simulink model "kepler_sgp4_test"  (Simulink 6.2)
settings: Solver=ode45  StartTime=0.0  StopTime=59516  RelTol=1e-3
undefined symbols (not defined in the file): onboardorbit, ONBOARDorbitECI
libraries: components_lib x4, simulink x2, sgp4_igrf_lib x2
settings Model: Creator=esch00  LastModifiedBy=rals
settings OptimizationCC: BlockReduction=off  BooleanDataType=off  InlineInvariantSignals=on
settings DebuggingCC: CheckSSInitialOutputMsg=off
settings HardwareCC: TargetUnknown=on

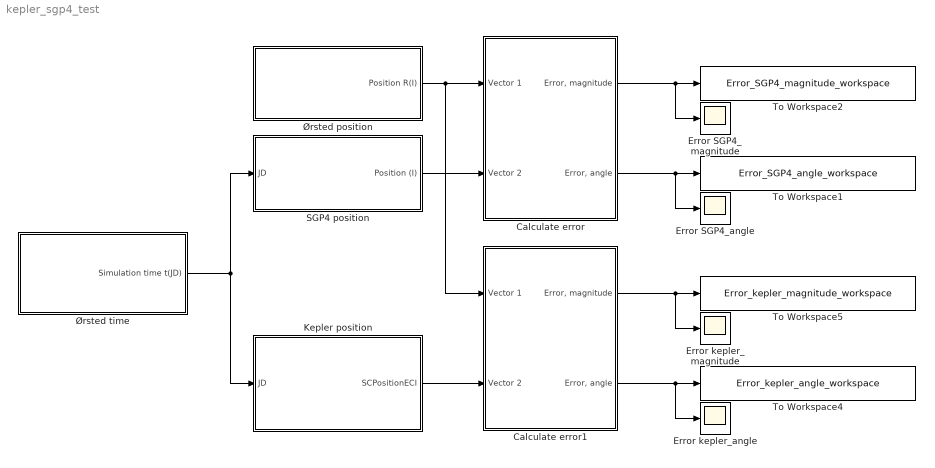
== system kepler_sgp4_test ==
  Calculate error : Subsystem
  Calculate error1 : Subsystem
  Error SGP4_angle : Scope
      settings: YMin=0  YMax=30000  SaveName=SGP4error1  DataFormat=Structure
  Error SGP4_magnitude : Scope
      settings: YMin=0  YMax=30000  SaveName=SGP4error  DataFormat=Structure
  Error kepler_angle : Scope
      settings: YMin=0  YMax=30000  SaveName=SGP4error2  DataFormat=Structure
  Error kepler_magnitude : Scope
      settings: YMin=0  YMax=30000  SaveName=SGP4error3  DataFormat=Structure
  Kepler position : Subsystem  AncestorBlock=onboardorbit/ONBOARDorbitECI
  SGP4 position : Subsystem  TreatAsAtomicUnit=on
  To Workspace1 : ToWorkspace  VariableName=Error_SGP4_angle_workspace  SampleTime=-1  SaveFormat=Array
  To Workspace2 : ToWorkspace  VariableName=Error_SGP4_magnitude_workspace  SampleTime=-1  SaveFormat=Array
  To Workspace4 : ToWorkspace  VariableName=Error_kepler_angle_workspace  SampleTime=-1  SaveFormat=Array
  To Workspace5 : ToWorkspace  VariableName=Error_kepler_magnitude_workspace  SampleTime=-1  SaveFormat=Array
  Ørsted position : Subsystem  TreatAsAtomicUnit=on
  Ørsted time : Subsystem  TreatAsAtomicUnit=on
  wires:
  Ørsted time/1(Simulation time t(JD)) -> Kepler position/1(JD), SGP4 position/1(JD)
  Ørsted position/1(Position R(I)) -> Calculate error/1(Vector 1), Calculate error1/1(Vector 1)
  SGP4 position/1(Position (I)) -> Calculate error/2(Vector 2)
  Calculate error/1("Error, magnitude") -> To Workspace2/1, Error SGP4_magnitude/1
  Calculate error/2("Error, angle") -> To Workspace1/1, Error SGP4_angle/1
  Calculate error1/1("Error, magnitude") -> To Workspace5/1, Error kepler_magnitude/1
  Calculate error1/2("Error, angle") -> To Workspace4/1, Error kepler_angle/1
  Kepler position/1(SCPositionECI) -> Calculate error1/2(Vector 2)

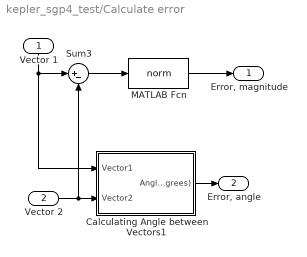
== system kepler_sgp4_test/Calculate error ==
  Vector 1 : Inport  Orientation=down  Port=1  LatchInput=off
  Vector 2 : Inport  Port=2  LatchInput=off
  Calculating Angle between Vectors1 : Subsystem
  MATLAB Fcn : MATLABFcn  MATLABFcn=norm
  Sum3 : Sum  Inputs=|+-  SaturateOnIntegerOverflow=on  InputSameDT=on
  "Error, magnitude" : Outport
  "Error, angle" : Outport  Port=2
  wires:
  Sum3/1 -> MATLAB Fcn/1
  Vector 2/1 -> Sum3/2, Calculating Angle between Vectors1/2(Vector2)
  Vector 1/1 -> Calculating Angle between Vectors1/1(Vector1), Sum3/1
  MATLAB Fcn/1 -> "Error, magnitude"/1
  Calculating Angle between Vectors1/1(Angle (Degrees)) -> "Error, angle"/1

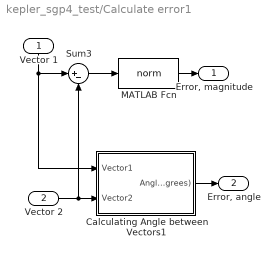
== system kepler_sgp4_test/Calculate error1 ==
  Vector 1 : Inport  Orientation=down  Port=1  LatchInput=off
  Vector 2 : Inport  Port=2  LatchInput=off
  Calculating Angle between Vectors1 : Subsystem
  MATLAB Fcn : MATLABFcn  MATLABFcn=norm
  Sum3 : Sum  Inputs=|+-  SaturateOnIntegerOverflow=on  InputSameDT=on
  "Error, magnitude" : Outport
  "Error, angle" : Outport  Port=2
  wires:
  Sum3/1 -> MATLAB Fcn/1
  Vector 2/1 -> Sum3/2, Calculating Angle between Vectors1/2(Vector2)
  Vector 1/1 -> Calculating Angle between Vectors1/1(Vector1), Sum3/1
  MATLAB Fcn/1 -> "Error, magnitude"/1
  Calculating Angle between Vectors1/1(Angle (Degrees)) -> "Error, angle"/1

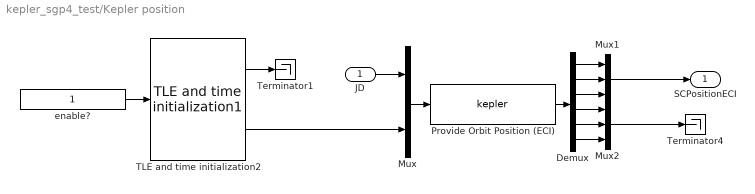
== system kepler_sgp4_test/Kepler position ==
  JD : Inport  Port=1  LatchInput=off
  Demux : Demux  Outputs=6
  Mux : Mux  Inputs=2
  Mux1 : Mux  Inputs=3
  Mux2 : Mux  Inputs=3
  Provide Orbit Position (ECI) : S-Function  FunctionName=kepler
  TLE and time initialization2 : sgp4_igrf_lib/Orbit and Magnetic field models/TLE and time initialization1  satname='Orsted'  YYDDD=02039  JulianDay=2452275.5+40.69255057  xndt2o=0.00002748*0  xndd6o=0  bstar=0.00071190  xincl=96.4788  xnodeo=112.1945  eo=0.0148615  omegao=71.6037  xmo=290.1241  xno=14.43891950  ts=1
  Terminator1 : Terminator
  Terminator4 : Terminator
  enable? : Constant
  SCPositionECI : Outport  InitialOutput=0
  wires:
  TLE and time initialization2/2 -> Mux/2
  JD/1 -> Mux/1
  Mux/1 -> Provide Orbit Position (ECI)/1
  Provide Orbit Position (ECI)/1 -> Demux/1
  Mux1/1 -> SCPositionECI/1
  Demux/1 -> Mux1/1
  Demux/2 -> Mux1/2
  Demux/3 -> Mux1/3
  Demux/4 -> Mux2/1
  Demux/5 -> Mux2/2
  Demux/6 -> Mux2/3
  Mux2/1 -> Terminator4/1
  TLE and time initialization2/1 -> Terminator1/1
  enable?/1 -> TLE and time initialization2/1

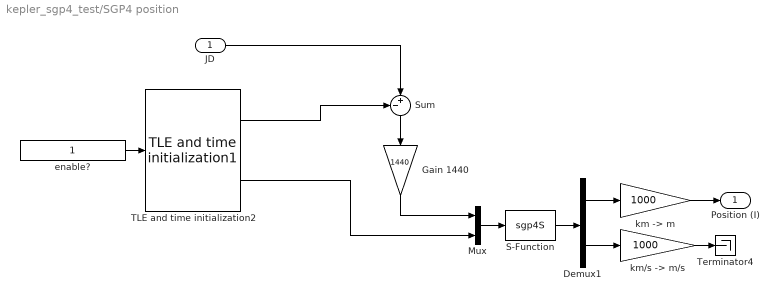
== system kepler_sgp4_test/SGP4 position ==
  JD : Inport  Port=1  LatchInput=off
  " S-Function" : S-Function  FunctionName=sgp4S
  Demux1 : Demux  Outputs=[3 3]
  Gain 1440 : Gain  Orientation=down  Gain=1440  SaturateOnIntegerOverflow=on
  Mux : Mux  Inputs=2
  Sum : Sum  Orientation=down  Inputs=-+|  SaturateOnIntegerOverflow=on  InputSameDT=on
  TLE and time initialization2 : sgp4_igrf_lib/Orbit and Magnetic field models/TLE and time initialization1  satname='Orsted'  YYDDD=02039  JulianDay=2452275.5+40.69255057  xndt2o=0.00002748*0  xndd6o=0  bstar=0.00071190  xincl=96.4788  xnodeo=112.1945  eo=0.0148615  omegao=71.6037  xmo=290.1241  xno=14.43891950  ts=1
  Terminator4 : Terminator
  enable? : Constant
  "km -> m" : Gain  Gain=1000  SaturateOnIntegerOverflow=on
  "km/s -> m/s" : Gain  Gain=1000  SaturateOnIntegerOverflow=on
  Position (I) : Outport  InitialOutput=0
  wires:
  JD/1 -> Sum/2
  "km -> m"/1 -> Position (I)/1
  "km/s -> m/s"/1 -> Terminator4/1
  Mux/1 -> " S-Function"/1
  " S-Function"/1 -> Demux1/1
  Demux1/2 -> "km/s -> m/s"/1
  Demux1/1 -> "km -> m"/1
  TLE and time initialization2/1 -> Sum/1
  Sum/1 -> Gain 1440/1
  Gain 1440/1 -> Mux/1
  TLE and time initialization2/2 -> Mux/2
  enable?/1 -> TLE and time initialization2/1

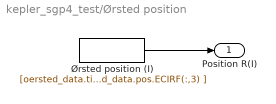
== system kepler_sgp4_test/Ørsted position ==
  Ørsted position (I) : FromWorkspace  VariableName=[oersted_data.time.sample_number oersted_data.pos.ECIRF(:,1) oersted_data.pos.ECIRF(:,2) oersted_data.pos.ECIRF(:,3) ]  SampleTime=1
  Position R(I) : Outport
  wires:
  Ørsted position (I)/1 -> Position R(I)/1

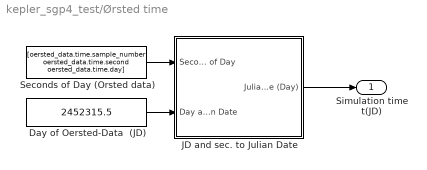
== system kepler_sgp4_test/Ørsted time ==
  Day of Oersted-Data  (JD) : Constant  Value=2452315.5
  JD and sec. to Julian Date : Subsystem
  Seconds of Day (Orsted data) : FromWorkspace  VariableName=[oersted_data.time.sample_number oersted_data.time.second oersted_data.time.day]  SampleTime=1
  Simulation time t(JD) : Outport
  wires:
  Seconds of Day (Orsted data)/1 -> JD and sec. to Julian Date/1(Second of Day)
  Day of Oersted-Data  (JD)/1 -> JD and sec. to Julian Date/2(Day as Julian Date)
  JD and sec. to Julian Date/1(Julian Date (Day)) -> Simulation time t(JD)/1

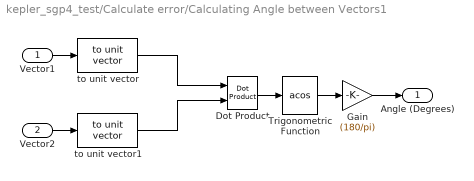
== system kepler_sgp4_test/Calculate error/Calculating Angle between Vectors1 ==
  Vector1 : Inport  Port=1  LatchInput=off
  Vector2 : Inport  Port=2  LatchInput=off
  Dot Product : simulink/Math Operations/Dot Product  InputSameDT=on  OutDataType=sfix(16)  OutScaling=2^-10  DoSatur=off
  Gain : Gain  Gain=(180/pi)  SaturateOnIntegerOverflow=on
  Trigonometric Function : Trigonometry  Operator=acos
  to unit vector : components_lib/Math utilities/Vector operations/to unit vector
  to unit vector1 : components_lib/Math utilities/Vector operations/to unit vector
  Angle (Degrees) : Outport
  wires:
  Gain/1 -> Angle (Degrees)/1
  Trigonometric Function/1 -> Gain/1
  Dot Product/1 -> Trigonometric Function/1
  Vector1/1 -> to unit vector/1
  Vector2/1 -> to unit vector1/1
  to unit vector/1 -> Dot Product/1
  to unit vector1/1 -> Dot Product/2

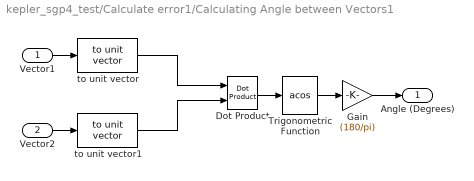
== system kepler_sgp4_test/Calculate error1/Calculating Angle between Vectors1 ==
  Vector1 : Inport  Port=1  LatchInput=off
  Vector2 : Inport  Port=2  LatchInput=off
  Dot Product : simulink/Math Operations/Dot Product  InputSameDT=on  OutDataType=sfix(16)  OutScaling=2^-10  DoSatur=off
  Gain : Gain  Gain=(180/pi)  SaturateOnIntegerOverflow=on
  Trigonometric Function : Trigonometry  Operator=acos
  to unit vector : components_lib/Math utilities/Vector operations/to unit vector
  to unit vector1 : components_lib/Math utilities/Vector operations/to unit vector
  Angle (Degrees) : Outport
  wires:
  Gain/1 -> Angle (Degrees)/1
  Trigonometric Function/1 -> Gain/1
  Dot Product/1 -> Trigonometric Function/1
  Vector1/1 -> to unit vector/1
  Vector2/1 -> to unit vector1/1
  to unit vector/1 -> Dot Product/1
  to unit vector1/1 -> Dot Product/2

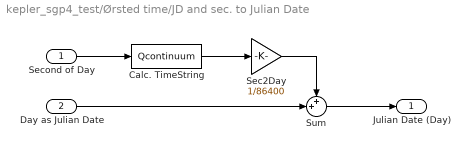
== system kepler_sgp4_test/Ørsted time/JD and sec. to Julian Date ==
  Second of Day : Inport  Port=1  LatchInput=off
  Day as Julian Date : Inport  Port=2  LatchInput=off
  Calc. TimeString : S-Function  FunctionName=Qcontinuum
  Sec2Day : Gain  Gain=1/86400  SaturateOnIntegerOverflow=on
  Sum : Sum  Inputs=++|  SaturateOnIntegerOverflow=on  InputSameDT=on
  Julian Date (Day) : Outport
  wires:
  Sum/1 -> Julian Date (Day)/1
  Second of Day/1 -> Calc. TimeString/1
  Day as Julian Date/1 -> Sum/2
  Sec2Day/1 -> Sum/1
  Calc. TimeString/1 -> Sec2Day/1
